simulink model "FxLMS_realtest"  (R2018a)
settings: Solver=FixedStepAuto  StartTime=0.0  StopTime=inf  RelTol=1e-3
libraries: audiosources x2, dspsnks4 x1
settings Model: Creator=gianc  LastModifiedBy=gianc
settings SolverCC: AutoInsertRateTranBlk=on
settings DataIOCC: LimitDataPoints=on  SaveOutput=off  SignalLogging=off  SaveTime=off
settings OptimizationCC: LifeSpan=inf
settings DebuggingCC: AlgebraicLoopMsg=error  SingleTaskRateTransMsg=error  AllowSymbolicDim=off  SFUnexpectedBacktrackingDiag=warning  SFNoUnconditionalDefaultTransitionDiag=warning  SFExecutionAtInitializationDiag=none
settings CodeAppCC: StateflowObjectComments=on
settings GRTTargetCC: TargetLangStandard=C89/C90 (ANSI)  GeneratePreprocessorConditionals=Disable all
settings ConfigComp: CovMetricSettings=dw  CovHtmlReporting=on  CovSaveCumulativeToWorkspaceVar=on  CovSaveSingleToWorkspaceVar=on  CovExternalEMLEnable=off  CovSFcnEnable=off

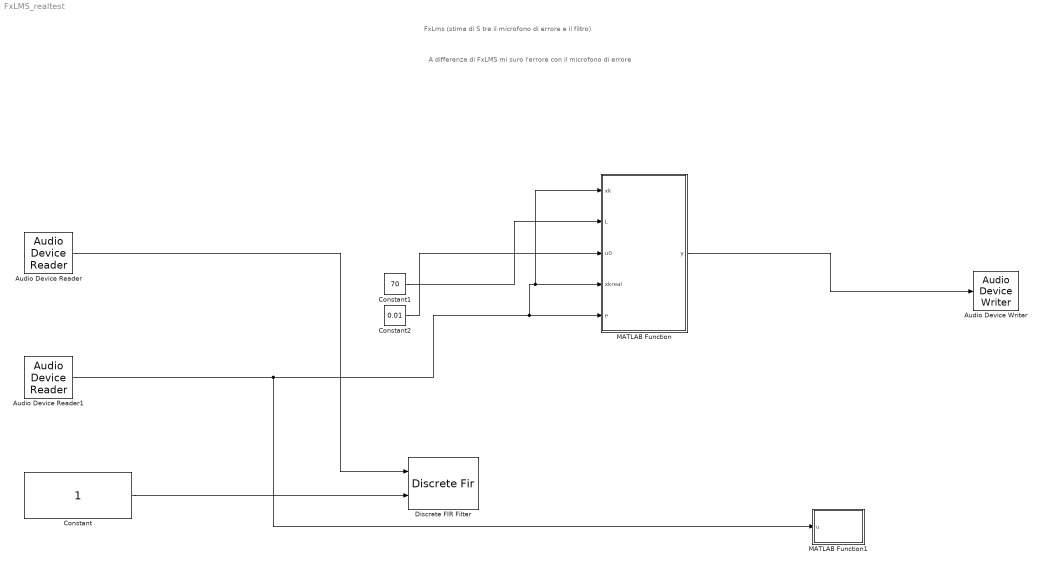
== system FxLMS_realtest ==
  note: A differenza di FxLMS mi suro l'errore con il microfono di errore
  note: FxLms (stima di S tra il microfono di errore e il filtro)
  Audio Device Reader : audiosources/Audio Device Reader  Driver=DirectSound  Device=Microfono (Realtek High Definition Audio)  SampleRate=8000  NumChannels=1  SamplesPerFrame=200  BitDepth=16-bit integer  NumBuffers=10  DefaultInputChannelMapping=on  InputChannelMapping=1:2  OutputNumOverrunSamples=off  OutputDataType=double  DriverIdx=1  DeviceWarnFlag=''
      settings: SourceProductName=Audio System Toolbox  SourceProductBaseCode=AU
  Audio Device Reader1 : audiosources/Audio Device Reader  Driver=DirectSound  Device=Microfono (2- USB PnP Sound Device)  SampleRate=8000  NumChannels=1  SamplesPerFrame=200  BitDepth=16-bit integer  NumBuffers=10  DefaultInputChannelMapping=on  InputChannelMapping=1:2  OutputNumOverrunSamples=off  OutputDataType=double  DriverIdx=1  DeviceWarnFlag=''
      settings: SourceProductName=Audio System Toolbox  SourceProductBaseCode=AU
  Audio Device Writer : dspsnks4/Audio Device Writer  Driver=DirectSound  Device=Default  InheritSampleRate=on  SampleRate=8000  BitDepth=16-bit integer  BufferSize=4096  NumBuffers=10  DefaultOutputChannelMapping=on  OutputChannelMapping=1:1  OutputNumUnderrunSamples=off  DriverIdx=1  DeviceWarnFlag=''
  Constant : Constant  VectorParams1D=off
  Constant1 : Constant  Value=70  VectorParams1D=off
  Constant2 : Constant  Value=0.01  VectorParams1D=off
  Discrete FIR Filter : DiscreteFir  CoefSource=Input port  InputProcessing=Columns as channels (frame based)
      settings: InputPortMap=u0,u1
  MATLAB Function : MATLAB Function  TreatAsAtomicUnit=on
  MATLAB Function1 : MATLAB Function  TreatAsAtomicUnit=on
  wires:
  Constant1/1 -> MATLAB Function/2(L)
  Constant/1 -> Discrete FIR Filter/2
  Constant2/1 -> MATLAB Function/3(u0)
  Audio Device Reader1/1 -> MATLAB Function1/1(u), MATLAB Function/1(xk), MATLAB Function/4(xkreal), MATLAB Function/5(e)
  Audio Device Reader/1 -> Discrete FIR Filter/1
  MATLAB Function/1(y) -> Audio Device Writer/1

== matlab function FxLMS_realtest/MATLAB Function1 ==
  data: u input
function fcn(u)
persistent t
if isempty(t)
    t=ones(200,1);
else
    t(1)=t(200)+1;
end

for i=1:199
    t(i+1)=t(i)+1;
end

hold on
plot(t,u,'g');

end

== matlab function FxLMS_realtest/MATLAB Function ==
  data: y output; xk input; L input; u0 input; xkreal input; e input
%y=output filter (anti noise)
%w=weights vector 1xL
%x=input vector 1xL
%xk=sampled input at time k
%d=wanted signal (ideal is x but we have d=P*x)

function y   = fxLMS(xk,L,u0,xkreal,e)

%global variables
[sizeD,~]=size(xk);
y=zeros(sizeD,1);
%yreal=zeros(sizeD,1);
u=u0;
%e=zeros(sizeD,1);
alpha=0.01;
persistent cnt
persistent x
persistent xreal
persistent w

for i=1:sizeD
    
if isempty(cnt)
    cnt=1;
else
    cnt=cnt+1;
end

if isempty(x)
    x=zeros(1,L);
end

if isempty(xreal)
    xreal=zeros(1,L);
end

if isempty(w)
    w=zeros(1,L);
end

%calculate u opt
if cnt<=L
    u=u0;
else
    if cnt==L
        u = max(u0,alpha/(xreal*(xreal')));
    else
        u = alpha/max(u/alpha,xreal*(xreal'));
    end
end
%LMS
xreal=[xkreal(i,1) xreal(1:(L-1))];%shift and add xkreal
x=[xk(i,1) x(1:(L-1))]; %shift and add xk (FIFO)
y(i)= w*(x'); %filter adapted
% yreal = convolution(y(i),s)
%[~,sizeS]=size(s);
%y_volatile=y(i)*ones(1,sizeS);
%yreal(i)=y_volatile*(s');
%e(i) = d(i,1)-yreal(i); % e measured with a sensor or estimated
w = w + u*xreal*e(i); %refresh w for the next iteration (LMS core)
end
end
